simulink model "Zigor_Model"  (R2012b)
settings: Solver=ode3  StartTime=0.0  StopTime=24*60*60  FixedStep=15*60  RelTol=1e-3
undefined symbols (not defined in the file or in its folder): DATA
settings Model: Creator=AW240643  LastModifiedBy=iepzugue
settings DataIOCC: SignalLoggingSaveFormat=ModelDataLogs
settings OptimizationCC: ExpressionDepthLimit=128
settings DebuggingCC: MultiTaskDSMMsg=warning  MultiTaskCondExecSysMsg=none  StateNameClashWarn=none  StrictBusMsg=None
settings RTWCC: IncludeERTFirstTime=on
settings CodeAppCC: CustomSymbolStrType=$N$R$M_T  InternalIdentifier=Shortened

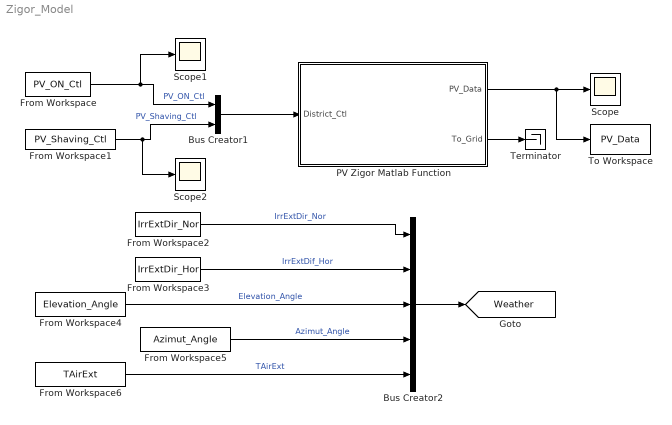
== system Zigor_Model ==
  Bus Creator1 : BusCreator  Inputs=2
  Bus Creator2 : BusCreator  Inputs=5
  From Workspace : FromWorkspace  VariableName=PV_ON_Ctl  SampleTime=0
  From Workspace1 : FromWorkspace  VariableName=PV_Shaving_Ctl  SampleTime=0
  From Workspace2 : FromWorkspace  VariableName=IrrExtDir_Nor  SampleTime=0
  From Workspace3 : FromWorkspace  VariableName=IrrExtDir_Hor  SampleTime=0
  From Workspace4 : FromWorkspace  VariableName=Elevation_Angle  SampleTime=0
  From Workspace5 : FromWorkspace  VariableName=Azimut_Angle  SampleTime=0
  From Workspace6 : FromWorkspace  VariableName=TAirExt  SampleTime=0
  PV Zigor Matlab Function : Subsystem
  Scope : Scope
  Scope1 : Scope
  Scope2 : Scope
      settings: SaveName=ScopeData2
  Terminator : Terminator
  To Workspace : ToWorkspace  VariableName=PV_Data  SampleTime=-1  SaveFormat=Structure With Time
  tag scope: Weather=global
  wires:
  Bus Creator1/1 -> PV Zigor Matlab Function/1(District_Ctl)
  From Workspace/1 -> Scope1/1, Bus Creator1/1  "PV_ON_Ctl"
  From Workspace1/1 -> Scope2/1, Bus Creator1/2  "PV_Shaving_Ctl"
  Bus Creator2/1 -> [Weather]
  From Workspace2/1 -> Bus Creator2/1  "IrrExtDir_Nor"
  From Workspace3/1 -> Bus Creator2/2  "IrrExtDif_Hor"
  From Workspace6/1 -> Bus Creator2/5  "TAirExt"
  From Workspace4/1 -> Bus Creator2/3  "Elevation_Angle"
  From Workspace5/1 -> Bus Creator2/4  "Azimut_Angle"
  PV Zigor Matlab Function/2(To_Grid) -> Terminator/1
  PV Zigor Matlab Function/1(PV_Data) -> To Workspace/1, Scope/1

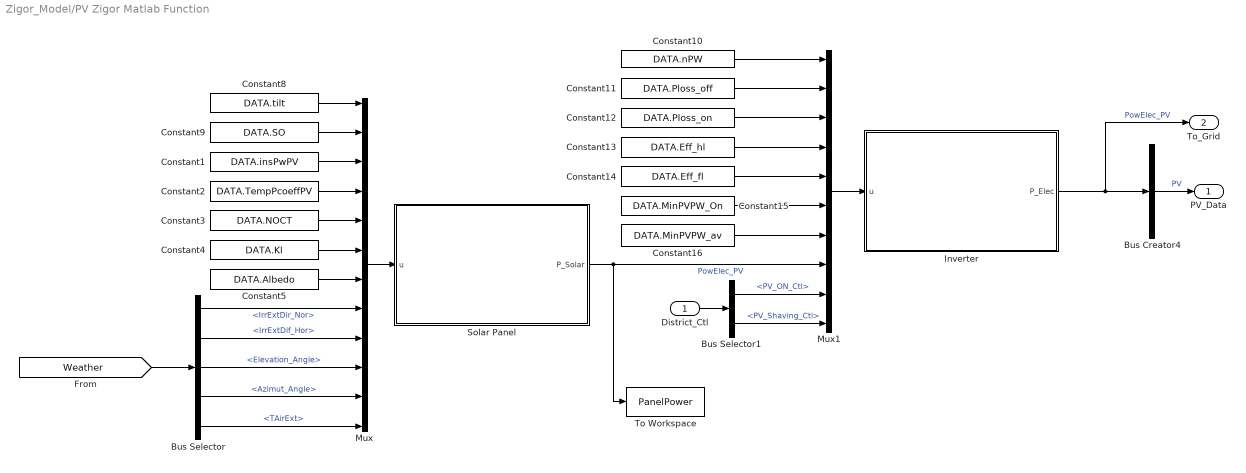
== system Zigor_Model/PV Zigor Matlab Function ==
  District_Ctl : Inport
  Bus Creator4 : BusCreator  Inputs=1
  Bus Selector : BusSelector  OutputSignals=IrrExtDir_Nor,IrrExtDif_Hor,Elevation_Angle,Azimut_Angle,TAirExt
  Bus Selector1 : BusSelector  OutputSignals=PV_ON_Ctl,PV_Shaving_Ctl
  Constant1 : Constant  Value=DATA.insPwPV
  Constant10 : Constant  Value=DATA.nPW
  Constant11 : Constant  Value=DATA.Ploss_off
  Constant12 : Constant  Value=DATA.Ploss_on
  Constant13 : Constant  Value=DATA.Eff_hl
  Constant14 : Constant  Value=DATA.Eff_fl
  Constant15 : Constant  Value=DATA.MinPVPW_On
  Constant16 : Constant  Value=DATA.MinPVPW_av
  Constant2 : Constant  Value=DATA.TempPcoeffPV
  Constant3 : Constant  Value=DATA.NOCT
  Constant4 : Constant  Value=DATA.Kl
  Constant5 : Constant  Value=DATA.Albedo
  Constant8 : Constant  Value=DATA.tilt
  Constant9 : Constant  Value=DATA.SO
  Inverter : MATLAB Function
  Mux : Mux  Inputs=12
  Mux1 : Mux  Inputs=10
  Solar Panel : MATLAB Function
  To Workspace : ToWorkspace  VariableName=PanelPower  SampleTime=-1  SaveFormat=Structure With Time
  PV_Data : Outport
  To_Grid : Outport  Port=2
  wires:
  Bus Creator4/1 -> PV_Data/1  "PV"
  District_Ctl/1 -> Bus Selector1/1
  Constant1/1 -> Mux/3
  Constant2/1 -> Mux/4
  Constant3/1 -> Mux/5
  Constant8/1 -> Mux/1
  Constant9/1 -> Mux/2
  Inverter/1(P_Elec) -> To_Grid/1, Bus Creator4/1  "PowElec_PV"
  Constant4/1 -> Mux/6
  [Weather] -> Bus Selector/1
  Mux/1 -> Solar Panel/1(u)
  Bus Selector/5 -> Mux/12  "<TAirExt>"
  Bus Selector/3 -> Mux/10  "<Elevation_Angle>"
  Bus Selector/1 -> Mux/8  "<IrrExtDir_Nor>"
  Mux1/1 -> Inverter/1(u)
  Bus Selector1/1 -> Mux1/9  "<PV_ON_Ctl>"
  Bus Selector1/2 -> Mux1/10  "<PV_Shaving_Ctl>"
  Solar Panel/1(P_Solar) -> To Workspace/1, Mux1/8  "PowElec_PV"
  Constant16/1 -> Mux1/7
  Constant15/1 -> Mux1/6
  Constant10/1 -> Mux1/1
  Constant11/1 -> Mux1/2
  Constant12/1 -> Mux1/3
  Constant13/1 -> Mux1/4
  Constant14/1 -> Mux1/5
  Constant5/1 -> Mux/7
  Bus Selector/2 -> Mux/9  "<IrrExtDif_Hor>"
  Bus Selector/4 -> Mux/11  "<Azimut_Angle>"

== matlab function Zigor_Model/PV Zigor Matlab Function/Inverter ==
  data: u input; P_Elec output
function P_Elec = Inverter(u)
Param.nPW = u(1);
Param.Eff.Ploss_off = u(2);
Param.Eff.Ploss_on = u(3);
Param.Eff.Eff_hl = u(4);
Param.Eff.Eff_fl = u(5);
Param.MinPVPW_On = u(6);
Param.MinPVPW_av = u(7);
PowSolar_PV = u(8);
PV_Ctl = u(9);
PV_Shaving_Ctl = u(10);


P_Elec = PowElec_PV(Param, PowSolar_PV, PV_Ctl, PV_Shaving_Ctl) ;

end

== matlab function Zigor_Model/PV Zigor Matlab Function/Solar Panel ==
  data: u input; P_Solar output size=1
function P_Solar = Solar_Panel(u)
Param.Orientation.tilt = u(1);
Param.Orientation.SO = u(2);
Param.insPwPV = u(3);
Param.TempPcoeffPV = u(4);
Param.NOCT = u(5);
Param.Kl = u(6);
Param.Albedo=u(7);
IrrDirect = u(8);
IrrDiffuse=u(9);
Elevation = u(10);
Azimuth = u(11);
Tair = u(12);

P_Solar = PowSolar_PV(Param, IrrDirect,IrrDiffuse, Elevation, Azimuth, Tair) ;

end
